simulink model "StaticSustainability2"  (R2020b)
settings: Solver=ode23tb  StartTime=0.0  StopTime=80  MaxStep=0.0001  RelTol=1e-3
undefined symbols (not defined in the file): D11, Delta, f_nom, H_gen, Kd_gen, R_gen, S_gen, V_gen, X_gen
libraries: powerlib x17, dspstat3 x16, powerlib_meascontrol x4, eeSequenceAnalyzer x4
settings Model: Creator=L  LastModifiedBy=New-life

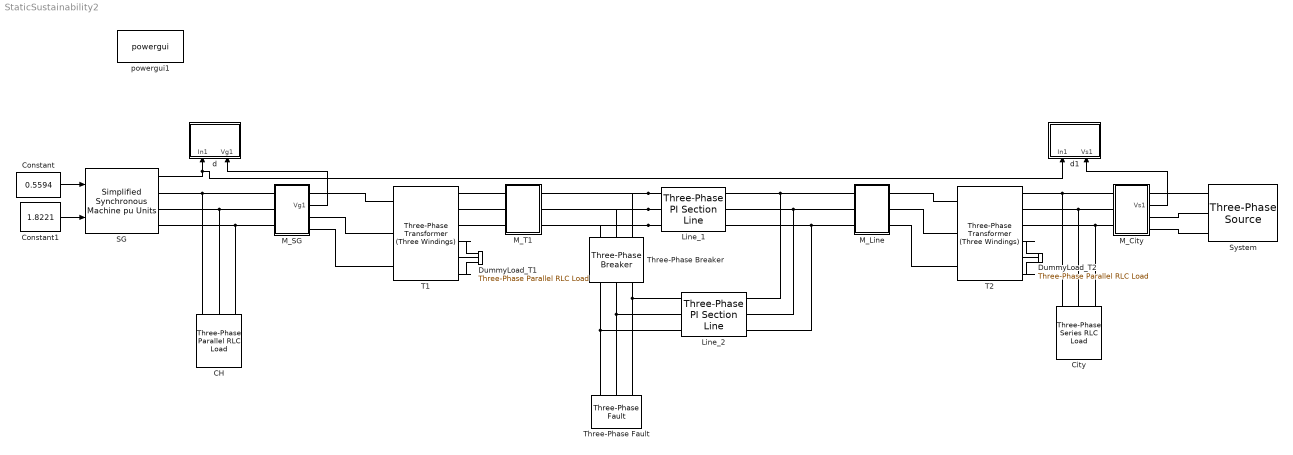
== system StaticSustainability2 ==
  CH : powerlib/Elements/Three-Phase Parallel RLC Load  LConnTagsString=A|B|C  Configuration=Y (grounded)  NominalVoltage=V_gen  Vabc=[1e3 1e3 1e3]  Vabcp=[1e3 1e3 1e3]  NominalFrequency=f_nom  UnbalancedPower=off  ActivePower=P_ch  InductivePower=Q_ch  CapacitivePower=0  Pabc=[10e3 9e3 11e3]  QLabc=[100 90 110]  QCabc=[100 90 110]  Pabcp=[10e3 9e3 11e3]  QLabcp=[100 90 110]  QCabcp=[100 90 110]  Measurements=None  LoadType=constant Z
  City : powerlib/Elements/Three-Phase Series RLC Load  LConnTagsString=A|B|C  Configuration=Y (grounded)  NominalVoltage=V_load  Vabc=[1e3 1e3 1e3]  Vabcp=[1e3 1e3 1e3]  NominalFrequency=f_nom  UnbalancedPower=off  ActivePower=P_load  InductivePower=Q_load  CapacitivePower=0  Pabc=[10e3 9e3 11e3]  QLabc=[100 90 110]  QCabc=[100 90 110]  Pabcp=[10e3 9e3 11e3]  QLabcp=[100 90 110]  QCabcp=[100 90 110]  Measurements=None  LoadType=constant Z
  Constant : Constant  Value=0.5594
  Constant1 : Constant  Value=1.8221
  DummyLoad_T1 : powerlib/Elements/Three-Phase Parallel RLC Load  LConnTagsString=A|B|C  Configuration=Y (grounded)  NominalVoltage=11e3  Vabc=[1e3 1e3 1e3]  Vabcp=[1e3 1e3 1e3]  NominalFrequency=50  UnbalancedPower=off  ActivePower=1  InductivePower=0  CapacitivePower=0  Pabc=[10e3 9e3 11e3]  QLabc=[100 90 110]  QCabc=[100 90 110]  Pabcp=[10e3 9e3 11e3]  QLabcp=[100 90 110]  QCabcp=[100 90 110]  Measurements=None  LoadType=constant Z
  DummyLoad_T2 : powerlib/Elements/Three-Phase Parallel RLC Load  LConnTagsString=A|B|C  Configuration=Y (grounded)  NominalVoltage=11e3  Vabc=[1e3 1e3 1e3]  Vabcp=[1e3 1e3 1e3]  NominalFrequency=50  UnbalancedPower=off  ActivePower=1  InductivePower=0  CapacitivePower=0  Pabc=[10e3 9e3 11e3]  QLabc=[100 90 110]  QCabc=[100 90 110]  Pabcp=[10e3 9e3 11e3]  QLabcp=[100 90 110]  QCabcp=[100 90 110]  Measurements=None  LoadType=constant Z
  Line_1 : powerlib/Elements/Three-Phase PI Section Line  LConnTagsString=a|b|c  RConnTagsString=A|B|C  Length=L_line  Frequency=f_nom  Resistances=R_line_vec  Inductances=L_line_vec  Capacitances=C_line_vec
  Line_2 : powerlib/Elements/Three-Phase PI Section Line  LConnTagsString=a|b|c  RConnTagsString=A|B|C  Length=L_line  Frequency=f_nom  Resistances=R_line_vec  Inductances=L_line_vec  Capacitances=C_line_vec
  M_City : Subsystem
      settings: PortSchema="{\"entries\":[{\"content\":{\"sides\":[{\"content\":{\"connectorIds\":[\"LConn1\",\"LConn2\",\"LConn3\"]},\"type\":\"ConnectorPlacement.EquallySpacedRectSide\",\"uuid\":\"295b92cf-ff7a-4ac6-8348-acc7c0051a63\"},{\"content\":{\"connectorIds\":[\"RConn1\",\"Out1\",\"RConn2\",\"RConn3\"],\"side\":\"RIGHT\"},\"type\":\"ConnectorPlacement.EquallySpacedRectSide\",\"uuid\":\"f69639b5-c750-459a-8cc2-14414b63acec\"},{\"content\":{\"connectorIds\":[],\"side\":\"TOP\"},\"type\":\"ConnectorPlacement.EquallySpacedRectSide\",\"uuid\":\"4a2635f6-db89-4dc3-8962-cf0290f1f42a\"},{\"content\":{\"connectorIds\":[],\"side\":\"HIDDEN\"},\"type\":\"ConnectorPlacement.EquallySpacedRectSide\",\"uuid\":\"64423351-ee21-4c85-9dc1-76181627d299\"}]},\"type\":\"ConnectorPlacement.EquallySpacedConnector\",\"uuid\":\"d8340770-254d-4d86-b26e-db3884cb831e\"}],\"packageUris\":[\"http://schema.mathworks.com/mf0/Connector/R2020b\"],\"version\":\"1.0\"}"
      settings: CopyFcn=|
      | % Получаем путь и имя нового (только что скопированного) блока
      | blockPath = gcb;
      | blockName = get_param(blockPath, 'Name');
      | 
      | % Ищем число в названии самой подсистемы (например, берем "2" из "Measure_2")
      | numStr = regexp(blockName, '\d+', 'match');
      | 
      | if ~isempty(numStr)
      |     newNum = numStr{end}; % Берем последнее найденное число
      | 
      |     % --- 1. Обновляем скрытые теги в Goto и From (радиочастоты) ---
      |     gotos = find_system(blockPath, 'LookUnderMasks', 'on', 'BlockType', 'Goto');
      |     froms = find_system(blockPath, 'LookUnderMasks', 'on', 'BlockType', 'From');
      | 
      |     for i = 1:length(gotos)
      |         oldTag = get_param(gotos{i}, 'GotoTag');
      |         set_param(gotos{i}, 'GotoTag', regexprep(oldTag, '\d+$', newNum));
      |     end
      |     for i = 1:length(froms)
      |         oldTag = get_param(froms{i}, 'GotoTag');
      |         set_param(froms{i}, 'GotoTag', regexprep(oldTag, '\d+$', newNum));
      |     end
      | 
      |     % --- 2. ПЕРЕИМЕНОВЫВАЕМ САМИ БЛОКИ (визуальные надписи UI0 -> UI1 и т.д.) ---
      |     % Ищем все элементы только внутри этой подсистемы
      |     internalBlocks = find_system(blockPath, 'SearchDepth', 1, 'LookUnderMasks', 'on');
      | 
      |     % Цикл начинаем с 2, так как 1-й элемент в списке - это сама папка подсистемы
      |     for i = 2:length(internalBlocks)
      |         oldName = get_param(internalBlocks{i}, 'Name');
      |         % Ищем цифру в конце имени и меняем на новую
      |         newName = regexprep(oldName, '\d+$', newNum);
      | 
      |         % Если имя изменилось, применяем его
      |         if ~strcmp(oldName, newName)
      |             try
      |                 set_param(internalBlocks{i}, 'Name', newName);
      |             catch
      |                 % Игнорируем ошибку, если вдруг такое имя уже случайно есть
      |             end
      |         end
      |     end
      | end
  M_SG : Subsystem
      settings: PortSchema="{\"entries\":[{\"content\":{\"sides\":[{\"content\":{\"connectorIds\":[\"LConn1\",\"LConn2\",\"LConn3\"]},\"type\":\"ConnectorPlacement.EquallySpacedRectSide\",\"uuid\":\"b0cf7806-418e-4dd9-bc8f-661d25e375f7\"},{\"content\":{\"connectorIds\":[\"RConn1\",\"Out1\",\"RConn2\",\"RConn3\"],\"side\":\"RIGHT\"},\"type\":\"ConnectorPlacement.EquallySpacedRectSide\",\"uuid\":\"097724a9-bedc-4684-9601-4545c29ec602\"},{\"content\":{\"connectorIds\":[],\"side\":\"TOP\"},\"type\":\"ConnectorPlacement.EquallySpacedRectSide\",\"uuid\":\"cba83770-cc70-4d4c-86bc-f56a9d8ba6d3\"},{\"content\":{\"connectorIds\":[],\"side\":\"HIDDEN\"},\"type\":\"ConnectorPlacement.EquallySpacedRectSide\",\"uuid\":\"7a6d872d-3c9e-483a-848d-3bbc65dc4943\"}]},\"type\":\"ConnectorPlacement.EquallySpacedConnector\",\"uuid\":\"3c4202e1-aed7-45b6-b37a-46ddcecd01e1\"}],\"packageUris\":[\"http://schema.mathworks.com/mf0/Connector/R2020b\"],\"version\":\"1.0\"}"
      settings: CopyFcn=|
      | % Получаем путь и имя нового (только что скопированного) блока
      | blockPath = gcb;
      | blockName = get_param(blockPath, 'Name');
      | 
      | % Ищем число в названии самой подсистемы (например, берем "2" из "Measure_2")
      | numStr = regexp(blockName, '\d+', 'match');
      | 
      | if ~isempty(numStr)
      |     newNum = numStr{end}; % Берем последнее найденное число
      | 
      |     % --- 1. Обновляем скрытые теги в Goto и From (радиочастоты) ---
      |     gotos = find_system(blockPath, 'LookUnderMasks', 'on', 'BlockType', 'Goto');
      |     froms = find_system(blockPath, 'LookUnderMasks', 'on', 'BlockType', 'From');
      | 
      |     for i = 1:length(gotos)
      |         oldTag = get_param(gotos{i}, 'GotoTag');
      |         set_param(gotos{i}, 'GotoTag', regexprep(oldTag, '\d+$', newNum));
      |     end
      |     for i = 1:length(froms)
      |         oldTag = get_param(froms{i}, 'GotoTag');
      |         set_param(froms{i}, 'GotoTag', regexprep(oldTag, '\d+$', newNum));
      |     end
      | 
      |     % --- 2. ПЕРЕИМЕНОВЫВАЕМ САМИ БЛОКИ (визуальные надписи UI0 -> UI1 и т.д.) ---
      |     % Ищем все элементы только внутри этой подсистемы
      |     internalBlocks = find_system(blockPath, 'SearchDepth', 1, 'LookUnderMasks', 'on');
      | 
      |     % Цикл начинаем с 2, так как 1-й элемент в списке - это сама папка подсистемы
      |     for i = 2:length(internalBlocks)
      |         oldName = get_param(internalBlocks{i}, 'Name');
      |         % Ищем цифру в конце имени и меняем на новую
      |         newName = regexprep(oldName, '\d+$', newNum);
      | 
      |         % Если имя изменилось, применяем его
      |         if ~strcmp(oldName, newName)
      |             try
      |                 set_param(internalBlocks{i}, 'Name', newName);
      |             catch
      |                 % Игнорируем ошибку, если вдруг такое имя уже случайно есть
      |             end
      |         end
      |     end
      | end
  M_T1 : Subsystem
      settings: CopyFcn=|
      | % Получаем путь и имя нового (только что скопированного) блока
      | blockPath = gcb;
      | blockName = get_param(blockPath, 'Name');
      | 
      | % Ищем число в названии самой подсистемы (например, берем "2" из "Measure_2")
      | numStr = regexp(blockName, '\d+', 'match');
      | 
      | if ~isempty(numStr)
      |     newNum = numStr{end}; % Берем последнее найденное число
      | 
      |     % --- 1. Обновляем скрытые теги в Goto и From (радиочастоты) ---
      |     gotos = find_system(blockPath, 'LookUnderMasks', 'on', 'BlockType', 'Goto');
      |     froms = find_system(blockPath, 'LookUnderMasks', 'on', 'BlockType', 'From');
      | 
      |     for i = 1:length(gotos)
      |         oldTag = get_param(gotos{i}, 'GotoTag');
      |         set_param(gotos{i}, 'GotoTag', regexprep(oldTag, '\d+$', newNum));
      |     end
      |     for i = 1:length(froms)
      |         oldTag = get_param(froms{i}, 'GotoTag');
      |         set_param(froms{i}, 'GotoTag', regexprep(oldTag, '\d+$', newNum));
      |     end
      | 
      |     % --- 2. ПЕРЕИМЕНОВЫВАЕМ САМИ БЛОКИ (визуальные надписи UI0 -> UI1 и т.д.) ---
      |     % Ищем все элементы только внутри этой подсистемы
      |     internalBlocks = find_system(blockPath, 'SearchDepth', 1, 'LookUnderMasks', 'on');
      | 
      |     % Цикл начинаем с 2, так как 1-й элемент в списке - это сама папка подсистемы
      |     for i = 2:length(internalBlocks)
      |         oldName = get_param(internalBlocks{i}, 'Name');
      |         % Ищем цифру в конце имени и меняем на новую
      |         newName = regexprep(oldName, '\d+$', newNum);
      | 
      |         % Если имя изменилось, применяем его
      |         if ~strcmp(oldName, newName)
      |             try
      |                 set_param(internalBlocks{i}, 'Name', newName);
      |             catch
      |                 % Игнорируем ошибку, если вдруг такое имя уже случайно есть
      |             end
      |         end
      |     end
      | end
  SG : powerlib/Machines/Simplified Synchronous Machine pu Units  ConnectionType=3-wire Y  MechanicalLoad=Mechanical power Pm  MeasurementBus=off  NominalParameters=[S_gen, V_gen, f_nom]  Mechanical=[H_gen, Kd_gen, 1]  InternalRL=[R_gen, X_gen]  InitialConditions=[0 44.3714 0.67318 0.67318 0.67318 -18.4954 -138.495 101.505]  IterativeDiscreteModel=Trapezoidal non iterative  TsBlock=-1  TsPowergui=0  LoadFlowParameters=[1,0,0,0,0]  Units=0  BusType=PQ  Pref=154.3e6  Qref=76.28e6  Qmin=-inf  Qmax=+inf  PLF=0  QLF=0
      settings: SourceProductBaseCode=PS
  System : powerlib/Electrical Sources/Three-Phase Source  InternalConnection=Yg  VoltagePhases=off  Voltage=(110000)*1.00459  PhaseAngle=0.37241  Voltage_phases=[25e3 25e3 25e3]/sqrt(3)  PhaseAngles_phases=[0 -120 +120]  Frequency=f_nom  NonIdealSource=on  SpecifyImpedance=on  Resistance=0.8929  Inductance=16.58e-3  ShortCircuitLevel=S_sc_sys  BaseVoltage=110000  XRratio=7  BusType=swing  Pref=10e3  Qref=0  Prefabc=[10e3, 10e3, 10e3]  Qrefabc=[0, 0, 0]  Qmin=-inf  Qmax=inf
  T1 : powerlib/Elements/Three-Phase Transformer (Three Windings)  Winding1Connection=Yg  Winding2Connection=Yg  Winding3Connection=Delta (D11)  CoreType=Three single-phase transformers  SetSaturation=off  Hysteresis=off  DataFile='hysteresis'  SetInitialFlux=off  Measurements=None  UNITS=pu  NominalPower=[250e6, 50]  Winding1=[10500, 0.0015, 0.055]  Winding2=[242000, 0.0015, 0.055]  Winding3=[11000, 0.001, 0.001]  Rm=500  Lm=500  L0=0.5  Saturation=[ 0,0 ; 0.0024,1.2 ; 1.0,1.52 ]  InitialFluxes=[0.8 -0.8 0.7]  BreakLoop=off  DiscreteSolver=Trapezoidal iterative  DataType=off  TransfoNumber=1
      settings: SourceProductBaseCode=PS
  T2 : powerlib/Elements/Three-Phase Transformer (Three Windings)  Winding1Connection=Yg  Winding2Connection=Yg  Winding3Connection=Delta (D11)  CoreType=Three single-phase transformers  SetSaturation=off  Hysteresis=off  DataFile='hysteresis'  SetInitialFlux=off  Measurements=None  UNITS=pu  NominalPower=[400e6, 50]  Winding1=[230000, 0.001, 0.115]  Winding2=[121000, 0.001, 0.001]  Winding3=[11000, 0.002, 0.205]  Rm=500  Lm=500  L0=0.5  Saturation=[ 0,0 ; 0.0024,1.2 ; 1.0,1.52 ]  InitialFluxes=[0.8 -0.8 0.7]  BreakLoop=off  DiscreteSolver=Trapezoidal iterative  DataType=off  TransfoNumber=1
      settings: SourceProductBaseCode=PS
  Three-Phase Breaker : powerlib/Elements/Three-Phase Breaker  InitialState=closed  SwitchA=on  SwitchB=on  SwitchC=on  SwitchTimes=[4.1]  External=off  BreakerResistance=0.01  SnubberResistance=1e6  SnubberCapacitance=inf  Measurements=None
  Three-Phase Fault : powerlib/Elements/Three-Phase Fault  InitialStates=0  FaultA=on  FaultB=on  FaultC=off  GroundFault=on  SwitchTimes=[4 4.1]  External=off  SwitchStatus=NaN  FaultResistance=0.001  GroundResistance=0.01  SnubberResistance=1e6  SnubberCapacitance=inf  Measurements=None
  d : Subsystem
  d1 : Subsystem
  powergui1 : powerlib/powergui  Priority=1  SimulationMode=Discrete  SampleTime=5e-5  frequency=50  Iterations=50  frequencyindice=50  Pbase=100e6  ErrMax=0.0001  UnitsV=kV  UnitsW=MW  buscounter=1  FunctionMessages=off  echomessages=off  EnableUseOfTLC=off  CurrentSourceSwitches=off  DisableSnubberDevices=off  DisableRonSwitches=off  DisableVfSwitches=off  DisplayEquations=off  AutomaticDiscreteSolvers=off  SolverType=Tustin/Backward Euler (TBE)  Interpol=off  ExternalGateDelay=off  methode=off  Ts=100  x0status=blocks  SPID=on  SwTol=0  HookPort=off  NonlinearTolerance=1e-4  nMaxIteration=100  ContinueOnMaxIteration=off  RestoreLinks=warning  ResistiveCurrentMeasurement=off  Frange=[0:2:500]  Ylog=off  Xlog=on  ShowGrid=off  save=off  variable=ZData  structure=0  ZoomFFT=off  StartTime=0.0  cycles=1  DisplayStyle=1  fundamental=60  FreqAxis=off  MaxFrequency=1000  frequencyindicesteady=1  RmsSteady=1  display=off
  М_Line : Subsystem
      settings: CopyFcn=|
      | % Получаем путь и имя нового (только что скопированного) блока
      | blockPath = gcb;
      | blockName = get_param(blockPath, 'Name');
      | 
      | % Ищем число в названии самой подсистемы (например, берем "2" из "Measure_2")
      | numStr = regexp(blockName, '\d+', 'match');
      | 
      | if ~isempty(numStr)
      |     newNum = numStr{end}; % Берем последнее найденное число
      | 
      |     % --- 1. Обновляем скрытые теги в Goto и From (радиочастоты) ---
      |     gotos = find_system(blockPath, 'LookUnderMasks', 'on', 'BlockType', 'Goto');
      |     froms = find_system(blockPath, 'LookUnderMasks', 'on', 'BlockType', 'From');
      | 
      |     for i = 1:length(gotos)
      |         oldTag = get_param(gotos{i}, 'GotoTag');
      |         set_param(gotos{i}, 'GotoTag', regexprep(oldTag, '\d+$', newNum));
      |     end
      |     for i = 1:length(froms)
      |         oldTag = get_param(froms{i}, 'GotoTag');
      |         set_param(froms{i}, 'GotoTag', regexprep(oldTag, '\d+$', newNum));
      |     end
      | 
      |     % --- 2. ПЕРЕИМЕНОВЫВАЕМ САМИ БЛОКИ (визуальные надписи UI0 -> UI1 и т.д.) ---
      |     % Ищем все элементы только внутри этой подсистемы
      |     internalBlocks = find_system(blockPath, 'SearchDepth', 1, 'LookUnderMasks', 'on');
      | 
      |     % Цикл начинаем с 2, так как 1-й элемент в списке - это сама папка подсистемы
      |     for i = 2:length(internalBlocks)
      |         oldName = get_param(internalBlocks{i}, 'Name');
      |         % Ищем цифру в конце имени и меняем на новую
      |         newName = regexprep(oldName, '\d+$', newNum);
      | 
      |         % Если имя изменилось, применяем его
      |         if ~strcmp(oldName, newName)
      |             try
      |                 set_param(internalBlocks{i}, 'Name', newName);
      |             catch
      |                 % Игнорируем ошибку, если вдруг такое имя уже случайно есть
      |             end
      |         end
      |     end
      | end
  wires:
  Constant/1 -> SG/1
  Constant1/1 -> SG/2
  SG/1 -> d1/1(In1), d/1(In1)
  M_SG/1(Vg1) -> d/2(Vg1)
  M_City/1(Vs1) -> d1/2(Vs1)
  connections:
  SG/RConn1 -- CH/LConn1 -- M_SG/LConn1
  SG/RConn2 -- CH/LConn2 -- M_SG/LConn2
  SG/RConn3 -- CH/LConn3 -- M_SG/LConn3
  T1/RConn1 -- M_T1/LConn1
  T1/RConn2 -- M_T1/LConn2
  T1/RConn3 -- M_T1/LConn3
  Line_1/LConn1 -- M_T1/RConn1 -- Three-Phase Breaker/LConn1
  Line_1/LConn2 -- M_T1/RConn2 -- Three-Phase Breaker/LConn2
  Line_1/LConn3 -- M_T1/RConn3 -- Three-Phase Breaker/LConn3
  Line_1/RConn1 -- Line_2/RConn1 -- М_Line/LConn1
  Line_1/RConn2 -- Line_2/RConn2 -- М_Line/LConn2
  Line_1/RConn3 -- Line_2/RConn3 -- М_Line/LConn3
  City/LConn1 -- M_City/LConn1 -- T2/RConn1
  City/LConn2 -- T2/RConn2 -- M_City/LConn2
  City/LConn3 -- T2/RConn3 -- M_City/LConn3
  T1/LConn2 -- M_SG/RConn2
  T1/LConn1 -- M_SG/RConn1
  М_Line/RConn2 -- T2/LConn2
  T2/LConn1 -- М_Line/RConn1
  T2/LConn3 -- М_Line/RConn3
  System/RConn3 -- M_City/RConn3
  System/RConn2 -- M_City/RConn2
  System/RConn1 -- M_City/RConn1
  M_SG/RConn3 -- T1/LConn3
  T1/RConn4 -- DummyLoad_T1/LConn1
  T1/RConn5 -- DummyLoad_T1/LConn2
  T1/RConn6 -- DummyLoad_T1/LConn3
  T2/RConn4 -- DummyLoad_T2/LConn1
  T2/RConn5 -- DummyLoad_T2/LConn2
  T2/RConn6 -- DummyLoad_T2/LConn3
  Three-Phase Fault/LConn3 -- Three-Phase Breaker/RConn3 -- Line_2/LConn3
  Three-Phase Fault/LConn2 -- Three-Phase Breaker/RConn2 -- Line_2/LConn2
  Three-Phase Fault/LConn1 -- Line_2/LConn1 -- Three-Phase Breaker/RConn1

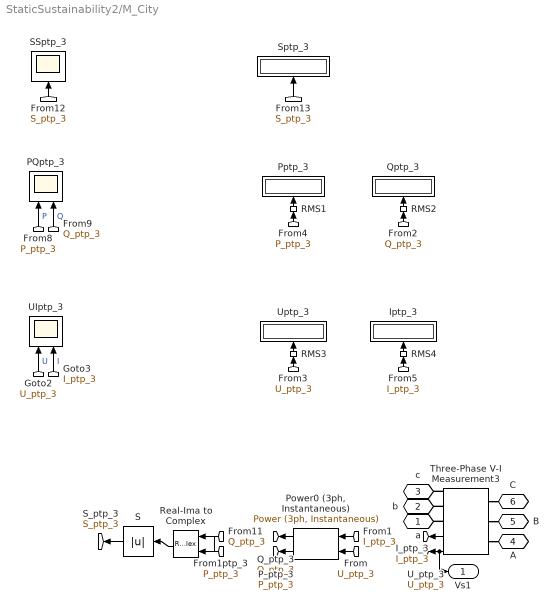
== system StaticSustainability2/M_City ==
  Iptp_3 : Display
      settings: Format=bank
  PQptp_3 : Scope  NumInputPorts=2
  "Power0 (3ph, Instantaneous)" : powerlib_meascontrol/Measurements/Power (3ph, Instantaneous)
  Pptp_3 : Display
      settings: Format=bank
  Qptp_3 : Display
      settings: Format=bank
  RMS{1..4} (4 alike) : dspstat3/RMS  run=off  directionMode=Each column  dimension=1  InputProcessing=Columns as channels (frame based)  reset_popup=None
  Real-Ima to Complex : RealImagToComplex
  S : Abs
  SSptp_3 : Scope
  Sptp_3 : Display
      settings: Format=bank
  Three-Phase V-I Measurement3 : powerlib/Measurements/Three-Phase V-I Measurement  VoltageMeasurement=phase-to-phase  SetLabelV=off  LabelV=Vabc  Vpu=off  VpuLL=off  CurrentMeasurement=yes  SetLabelI=off  LabelI=Iabc  Ipu=off  Pbase=100e6  Vbase=500e3  OutputType=Complex  PhasorSimulation=off  PSBequivalent=0
  UIptp_3 : Scope  NumInputPorts=2
  Uptp_3 : Display
      settings: Format=bank
  a : PMIOPort  Side=Right
  b : PMIOPort  Port=2  Side=Right
  c : PMIOPort  Port=3  Side=Right
  A : PMIOPort  Port=4  Side=Left
  B : PMIOPort  Port=5  Side=Left
  C : PMIOPort  Port=6  Side=Left
  Vs1 : Outport
  tag scope: I_ptp_3=global, P_ptp_3=global, Q_ptp_3=global, S_ptp_3=global, U_ptp_3=global
  wires:
  S/1 -> [S_ptp_3]
  Real-Ima to Complex/1 -> S/1
  [S_ptp_3] -> Sptp_3/1
  [S_ptp_3] -> SSptp_3/1
  [P_ptp_3] -> RMS1/1
  RMS1/1 -> Pptp_3/1
  RMS2/1 -> Qptp_3/1
  [U_ptp_3] -> RMS3/1
  RMS3/1 -> Uptp_3/1
  [P_ptp_3] -> Real-Ima to Complex/1
  [Q_ptp_3] -> RMS2/1
  [I_ptp_3] -> RMS4/1
  RMS4/1 -> Iptp_3/1
  [U_ptp_3] -> UIptp_3/1  "U"
  Three-Phase V-I Measurement3/1 -> Vs1/1, [U_ptp_3]
  [Q_ptp_3] -> Real-Ima to Complex/2
  Three-Phase V-I Measurement3/2 -> [I_ptp_3]
  [U_ptp_3] -> "Power0 (3ph, Instantaneous)"/1
  [I_ptp_3] -> "Power0 (3ph, Instantaneous)"/2
  "Power0 (3ph, Instantaneous)"/2 -> [Q_ptp_3]
  "Power0 (3ph, Instantaneous)"/1 -> [P_ptp_3]
  [I_ptp_3] -> UIptp_3/2  "I"
  [P_ptp_3] -> PQptp_3/1  "P"
  [Q_ptp_3] -> PQptp_3/2  "Q"
  connections:
  Three-Phase V-I Measurement3/LConn1 -- A/RConn1
  Three-Phase V-I Measurement3/RConn1 -- a/RConn1
  Three-Phase V-I Measurement3/LConn2 -- B/RConn1
  Three-Phase V-I Measurement3/LConn3 -- C/RConn1
  Three-Phase V-I Measurement3/RConn3 -- c/RConn1
  Three-Phase V-I Measurement3/RConn2 -- b/RConn1

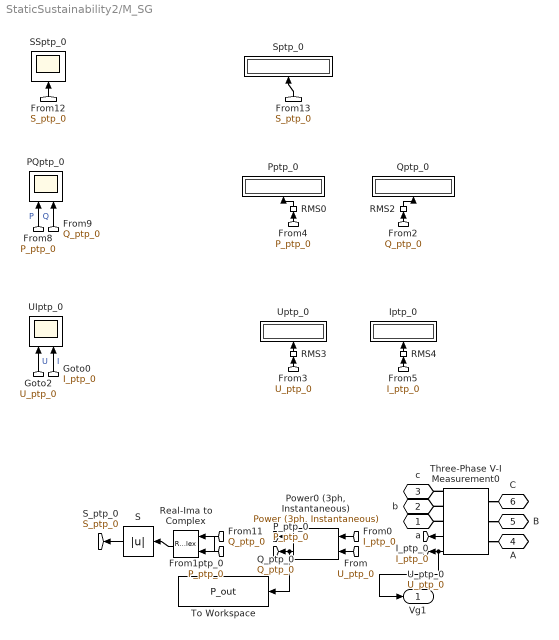
== system StaticSustainability2/M_SG ==
  Iptp_0 : Display
      settings: Format=bank
  PQptp_0 : Scope  NumInputPorts=2
  "Power0 (3ph, Instantaneous)" : powerlib_meascontrol/Measurements/Power (3ph, Instantaneous)
  Pptp_0 : Display
      settings: Format=bank
  Qptp_0 : Display
      settings: Format=bank
  RMS{0,2..4} (4 alike) : dspstat3/RMS  run=off  directionMode=Each column  dimension=1  InputProcessing=Columns as channels (frame based)  reset_popup=None
  Real-Ima to Complex : RealImagToComplex
  S : Abs
  SSptp_0 : Scope
  Sptp_0 : Display
      settings: Format=bank
  Three-Phase V-I Measurement0 : powerlib/Measurements/Three-Phase V-I Measurement  VoltageMeasurement=phase-to-phase  SetLabelV=off  LabelV=Vabc  Vpu=off  VpuLL=off  CurrentMeasurement=yes  SetLabelI=off  LabelI=Iabc  Ipu=off  Pbase=100e6  Vbase=500e3  OutputType=Complex  PhasorSimulation=off  PSBequivalent=0
  To Workspace : ToWorkspace  VariableName=P_out  SampleTime=-1
  UIptp_0 : Scope  NumInputPorts=2
  Uptp_0 : Display
      settings: Format=bank
  a : PMIOPort  Side=Right
  b : PMIOPort  Port=2  Side=Right
  c : PMIOPort  Port=3  Side=Right
  A : PMIOPort  Port=4  Side=Left
  B : PMIOPort  Port=5  Side=Left
  C : PMIOPort  Port=6  Side=Left
  Vg1 : Outport
  tag scope: I_ptp_0=global, P_ptp_0=global, Q_ptp_0=global, S_ptp_0=global, U_ptp_0=global
  wires:
  [Q_ptp_0] -> PQptp_0/2  "Q"
  [P_ptp_0] -> PQptp_0/1  "P"
  [I_ptp_0] -> UIptp_0/2  "I"
  "Power0 (3ph, Instantaneous)"/1 -> To Workspace/1, [P_ptp_0]
  "Power0 (3ph, Instantaneous)"/2 -> [Q_ptp_0]
  [I_ptp_0] -> "Power0 (3ph, Instantaneous)"/2
  [U_ptp_0] -> "Power0 (3ph, Instantaneous)"/1
  Three-Phase V-I Measurement0/2 -> [I_ptp_0]
  [Q_ptp_0] -> Real-Ima to Complex/2
  Three-Phase V-I Measurement0/1 -> Vg1/1, [U_ptp_0]
  [U_ptp_0] -> UIptp_0/1  "U"
  RMS4/1 -> Iptp_0/1
  [I_ptp_0] -> RMS4/1
  [Q_ptp_0] -> RMS2/1
  [P_ptp_0] -> Real-Ima to Complex/1
  RMS3/1 -> Uptp_0/1
  [U_ptp_0] -> RMS3/1
  RMS2/1 -> Qptp_0/1
  RMS0/1 -> Pptp_0/1
  [P_ptp_0] -> RMS0/1
  [S_ptp_0] -> SSptp_0/1
  [S_ptp_0] -> Sptp_0/1
  Real-Ima to Complex/1 -> S/1
  S/1 -> [S_ptp_0]
  connections:
  Three-Phase V-I Measurement0/RConn2 -- b/RConn1
  Three-Phase V-I Measurement0/RConn3 -- c/RConn1
  Three-Phase V-I Measurement0/LConn3 -- C/RConn1
  Three-Phase V-I Measurement0/LConn2 -- B/RConn1
  Three-Phase V-I Measurement0/RConn1 -- a/RConn1
  Three-Phase V-I Measurement0/LConn1 -- A/RConn1

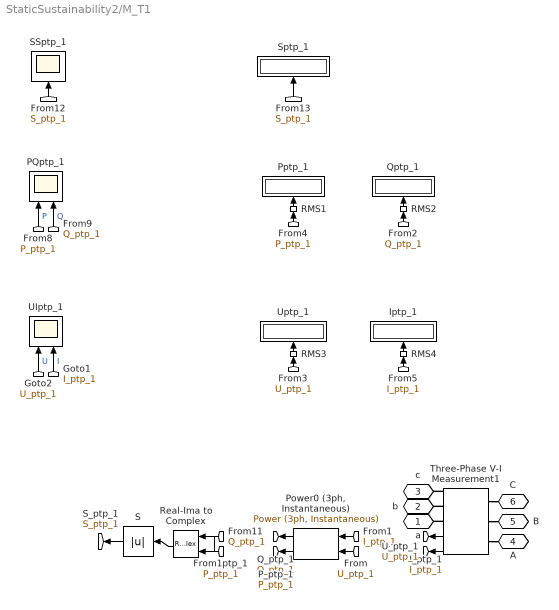
== system StaticSustainability2/M_T1 ==
  Iptp_1 : Display
      settings: Format=bank
  PQptp_1 : Scope  NumInputPorts=2
  "Power0 (3ph, Instantaneous)" : powerlib_meascontrol/Measurements/Power (3ph, Instantaneous)
  Pptp_1 : Display
      settings: Format=bank
  Qptp_1 : Display
      settings: Format=bank
  RMS{1..4} (4 alike) : dspstat3/RMS  run=off  directionMode=Each column  dimension=1  InputProcessing=Columns as channels (frame based)  reset_popup=None
  Real-Ima to Complex : RealImagToComplex
  S : Abs
  SSptp_1 : Scope
  Sptp_1 : Display
      settings: Format=bank
  Three-Phase V-I Measurement1 : powerlib/Measurements/Three-Phase V-I Measurement  VoltageMeasurement=phase-to-phase  SetLabelV=off  LabelV=Vabc  Vpu=off  VpuLL=off  CurrentMeasurement=yes  SetLabelI=off  LabelI=Iabc  Ipu=off  Pbase=100e6  Vbase=500e3  OutputType=Complex  PhasorSimulation=off  PSBequivalent=0
  UIptp_1 : Scope  NumInputPorts=2
  Uptp_1 : Display
      settings: Format=bank
  a : PMIOPort  Side=Right
  b : PMIOPort  Port=2  Side=Right
  c : PMIOPort  Port=3  Side=Right
  A : PMIOPort  Port=4  Side=Left
  B : PMIOPort  Port=5  Side=Left
  C : PMIOPort  Port=6  Side=Left
  tag scope: I_ptp_1=global, P_ptp_1=global, Q_ptp_1=global, S_ptp_1=global, U_ptp_1=global
  wires:
  S/1 -> [S_ptp_1]
  Real-Ima to Complex/1 -> S/1
  [S_ptp_1] -> Sptp_1/1
  [S_ptp_1] -> SSptp_1/1
  [P_ptp_1] -> RMS1/1
  RMS1/1 -> Pptp_1/1
  RMS2/1 -> Qptp_1/1
  [U_ptp_1] -> RMS3/1
  RMS3/1 -> Uptp_1/1
  [P_ptp_1] -> Real-Ima to Complex/1
  [Q_ptp_1] -> RMS2/1
  [I_ptp_1] -> RMS4/1
  RMS4/1 -> Iptp_1/1
  [U_ptp_1] -> UIptp_1/1  "U"
  Three-Phase V-I Measurement1/1 -> [U_ptp_1]
  [Q_ptp_1] -> Real-Ima to Complex/2
  Three-Phase V-I Measurement1/2 -> [I_ptp_1]
  [U_ptp_1] -> "Power0 (3ph, Instantaneous)"/1
  [I_ptp_1] -> "Power0 (3ph, Instantaneous)"/2
  "Power0 (3ph, Instantaneous)"/2 -> [Q_ptp_1]
  "Power0 (3ph, Instantaneous)"/1 -> [P_ptp_1]
  [I_ptp_1] -> UIptp_1/2  "I"
  [P_ptp_1] -> PQptp_1/1  "P"
  [Q_ptp_1] -> PQptp_1/2  "Q"
  connections:
  Three-Phase V-I Measurement1/LConn1 -- A/RConn1
  Three-Phase V-I Measurement1/RConn1 -- a/RConn1
  Three-Phase V-I Measurement1/LConn2 -- B/RConn1
  Three-Phase V-I Measurement1/LConn3 -- C/RConn1
  Three-Phase V-I Measurement1/RConn3 -- c/RConn1
  Three-Phase V-I Measurement1/RConn2 -- b/RConn1

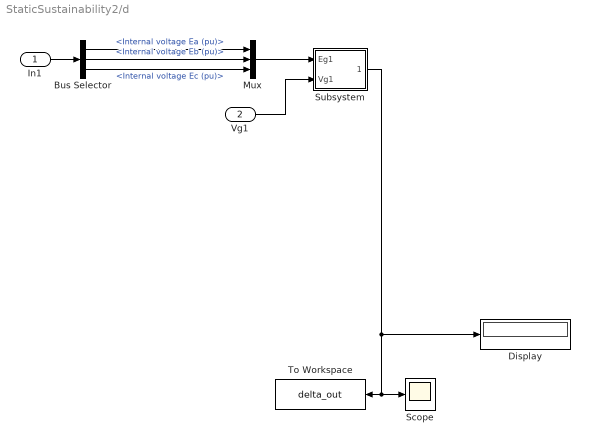
== system StaticSustainability2/d ==
  In1 : Inport
  Vg1 : Inport  Port=2
  Bus Selector : BusSelector  OutputSignals=Internal voltage Ea (pu),Internal voltage Eb (pu),Internal voltage Ec (pu)
  Display : Display
  Mux : Mux  Inputs=3
  Scope : Scope
  Subsystem : Subsystem
  To Workspace : ToWorkspace  VariableName=delta_out  SampleTime=-1
  wires:
  Bus Selector/3 -> Mux/3  "<Internal voltage Ec (pu)>"
  Bus Selector/2 -> Mux/2  "<Internal voltage Eb (pu)>"
  Bus Selector/1 -> Mux/1  "<Internal voltage Ea (pu)>"
  In1/1 -> Bus Selector/1
  Subsystem/1(Delta) -> Display/1, Scope/1, To Workspace/1
  Mux/1 -> Subsystem/1(Eg1)
  Vg1/1 -> Subsystem/2(Vg1)

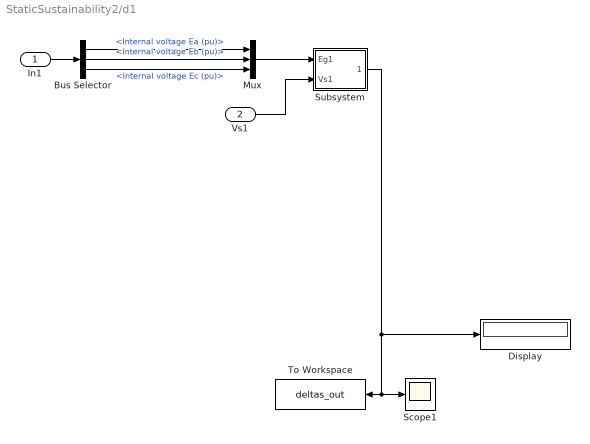
== system StaticSustainability2/d1 ==
  In1 : Inport
  Vs1 : Inport  Port=2
  Bus Selector : BusSelector  OutputSignals=Internal voltage Ea (pu),Internal voltage Eb (pu),Internal voltage Ec (pu)
  Display : Display
  Mux : Mux  Inputs=3
  Scope1 : Scope
  Subsystem : Subsystem
  To Workspace : ToWorkspace  VariableName=deltas_out  SampleTime=-1
  wires:
  Vs1/1 -> Subsystem/2(Vs1)
  Mux/1 -> Subsystem/1(Eg1)
  Subsystem/1(Delta) -> Scope1/1, To Workspace/1, Display/1
  In1/1 -> Bus Selector/1
  Bus Selector/1 -> Mux/1  "<Internal voltage Ea (pu)>"
  Bus Selector/2 -> Mux/2  "<Internal voltage Eb (pu)>"
  Bus Selector/3 -> Mux/3  "<Internal voltage Ec (pu)>"

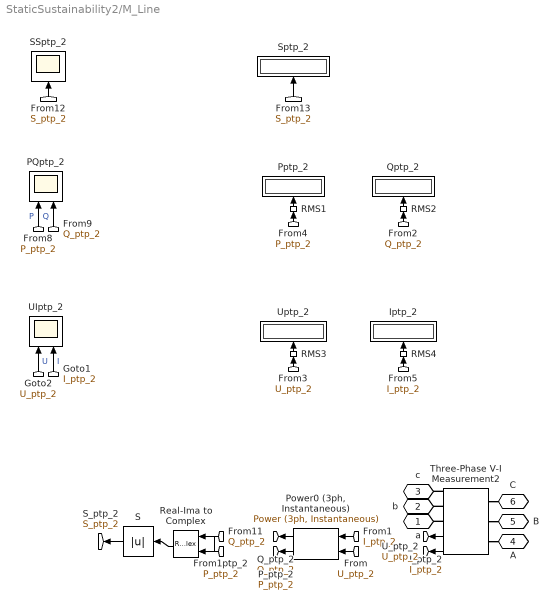
== system StaticSustainability2/М_Line ==
  Iptp_2 : Display
      settings: Format=bank
  PQptp_2 : Scope  NumInputPorts=2
  "Power0 (3ph, Instantaneous)" : powerlib_meascontrol/Measurements/Power (3ph, Instantaneous)
  Pptp_2 : Display
      settings: Format=bank
  Qptp_2 : Display
      settings: Format=bank
  RMS{1..4} (4 alike) : dspstat3/RMS  run=off  directionMode=Each column  dimension=1  InputProcessing=Columns as channels (frame based)  reset_popup=None
  Real-Ima to Complex : RealImagToComplex
  S : Abs
  SSptp_2 : Scope
  Sptp_2 : Display
      settings: Format=bank
  Three-Phase V-I Measurement2 : powerlib/Measurements/Three-Phase V-I Measurement  VoltageMeasurement=phase-to-phase  SetLabelV=off  LabelV=Vabc  Vpu=off  VpuLL=off  CurrentMeasurement=yes  SetLabelI=off  LabelI=Iabc  Ipu=off  Pbase=100e6  Vbase=500e3  OutputType=Complex  PhasorSimulation=off  PSBequivalent=0
  UIptp_2 : Scope  NumInputPorts=2
  Uptp_2 : Display
      settings: Format=bank
  a : PMIOPort  Side=Right
  b : PMIOPort  Port=2  Side=Right
  c : PMIOPort  Port=3  Side=Right
  A : PMIOPort  Port=4  Side=Left
  B : PMIOPort  Port=5  Side=Left
  C : PMIOPort  Port=6  Side=Left
  tag scope: I_ptp_2=global, P_ptp_2=global, Q_ptp_2=global, S_ptp_2=global, U_ptp_2=global
  wires:
  [Q_ptp_2] -> PQptp_2/2  "Q"
  [P_ptp_2] -> PQptp_2/1  "P"
  [I_ptp_2] -> UIptp_2/2  "I"
  "Power0 (3ph, Instantaneous)"/1 -> [P_ptp_2]
  "Power0 (3ph, Instantaneous)"/2 -> [Q_ptp_2]
  [I_ptp_2] -> "Power0 (3ph, Instantaneous)"/2
  [U_ptp_2] -> "Power0 (3ph, Instantaneous)"/1
  Three-Phase V-I Measurement2/2 -> [I_ptp_2]
  [Q_ptp_2] -> Real-Ima to Complex/2
  Three-Phase V-I Measurement2/1 -> [U_ptp_2]
  [U_ptp_2] -> UIptp_2/1  "U"
  RMS4/1 -> Iptp_2/1
  [I_ptp_2] -> RMS4/1
  [Q_ptp_2] -> RMS2/1
  [P_ptp_2] -> Real-Ima to Complex/1
  RMS3/1 -> Uptp_2/1
  [U_ptp_2] -> RMS3/1
  RMS2/1 -> Qptp_2/1
  RMS1/1 -> Pptp_2/1
  [P_ptp_2] -> RMS1/1
  [S_ptp_2] -> SSptp_2/1
  [S_ptp_2] -> Sptp_2/1
  Real-Ima to Complex/1 -> S/1
  S/1 -> [S_ptp_2]
  connections:
  Three-Phase V-I Measurement2/RConn2 -- b/RConn1
  Three-Phase V-I Measurement2/RConn3 -- c/RConn1
  Three-Phase V-I Measurement2/LConn3 -- C/RConn1
  Three-Phase V-I Measurement2/LConn2 -- B/RConn1
  Three-Phase V-I Measurement2/RConn1 -- a/RConn1
  Three-Phase V-I Measurement2/LConn1 -- A/RConn1

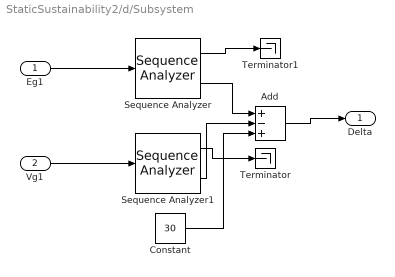
== system StaticSustainability2/d/Subsystem ==
  Eg1 : Inport
  Vg1 : Inport  Port=2
  Add : Sum  Inputs=+-+
  Constant : Constant  Value=30
  Sequence Analyzer : eeSequenceAnalyzer/Sequence Analyzer  VariantControl=Variant1  LabelModeActiveChoice=Continuous  F=50  K=[1]  Seq=Positive  Ts=0
      settings: SourceProductBaseCode=PS
  Sequence Analyzer1 : eeSequenceAnalyzer/Sequence Analyzer  VariantControl=Variant1  LabelModeActiveChoice=Continuous  F=50  K=[1]  Seq=Positive  Ts=0
      settings: SourceProductBaseCode=PS
  Terminator : Terminator
  Terminator1 : Terminator
  Delta : Outport
  wires:
  Sequence Analyzer/2 -> Add/1
  Sequence Analyzer1/2 -> Add/2
  Add/1 -> Delta/1
  Sequence Analyzer1/1 -> Terminator/1
  Sequence Analyzer/1 -> Terminator1/1
  Vg1/1 -> Sequence Analyzer1/1
  Eg1/1 -> Sequence Analyzer/1
  Constant/1 -> Add/3

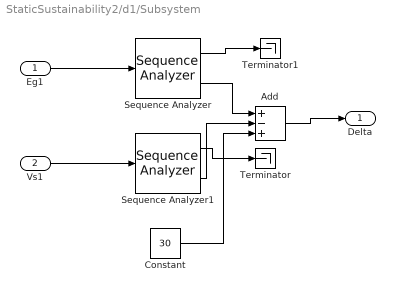
== system StaticSustainability2/d1/Subsystem ==
  Eg1 : Inport
  Vs1 : Inport  Port=2
  Add : Sum  Inputs=+-+
  Constant : Constant  Value=30
  Sequence Analyzer : eeSequenceAnalyzer/Sequence Analyzer  VariantControl=Variant1  LabelModeActiveChoice=Continuous  F=50  K=[1]  Seq=Positive  Ts=0
      settings: SourceProductBaseCode=PS
  Sequence Analyzer1 : eeSequenceAnalyzer/Sequence Analyzer  VariantControl=Variant1  LabelModeActiveChoice=Continuous  F=50  K=[1]  Seq=Positive  Ts=0
      settings: SourceProductBaseCode=PS
  Terminator : Terminator
  Terminator1 : Terminator
  Delta : Outport
  wires:
  Eg1/1 -> Sequence Analyzer/1
  Vs1/1 -> Sequence Analyzer1/1
  Sequence Analyzer/1 -> Terminator1/1
  Sequence Analyzer1/1 -> Terminator/1
  Add/1 -> Delta/1
  Sequence Analyzer1/2 -> Add/2
  Sequence Analyzer/2 -> Add/1
  Constant/1 -> Add/3
